simulink subsystem "ES"  (R2024a)
settings: Solver=VariableStepAuto  StartTime=0.0  StopTime=100.0  RelTol=1e-3
settings Model: DefaultTestHarness=ES_Harness1  Creator=nevil  LastModifiedBy=nevil

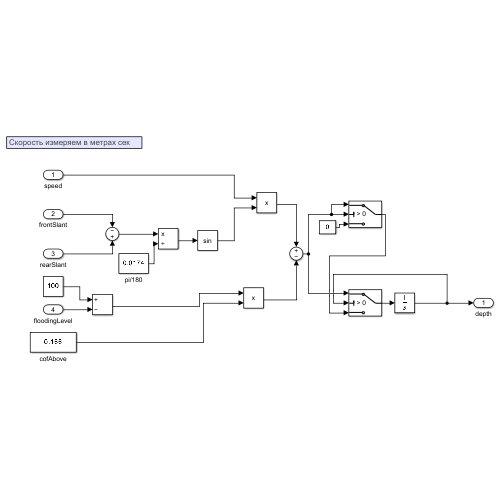
[thumbnail: Simulink's stored preview of the top-level diagram]
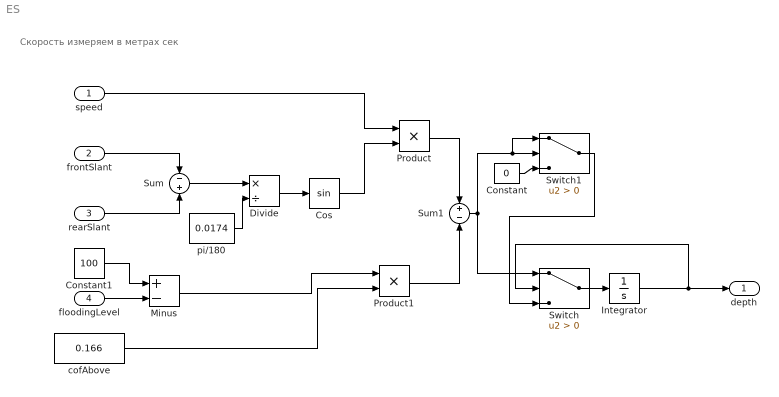
== system ES ==
  note: Скорость измеряем в метрах сек
  speed : Inport
  frontSlant : Inport  Port=2
  rearSlant : Inport  Port=3
  floodingLevel : Inport  Port=4
  Constant : Constant  Value=0
  Constant1 : Constant  Value=100
  Cos : Trigonometry
  Divide : Product  Inputs=*/
  Integrator : Integrator
  Minus : Sum  Inputs=+-
  Product : Product
  Product1 : Product
  Sum : Sum  Inputs=-|+
  Sum1 : Sum  Inputs=+|-
  Switch : Switch  Criteria=u2 > Threshold  SaturateOnIntegerOverflow=off  InputSameDT=off
  Switch1 : Switch  Criteria=u2 > Threshold  SaturateOnIntegerOverflow=off  InputSameDT=off
  cofAbove : Constant  Value=0.166
  pi/180 : Constant  Value=0.0174
  depth : Outport
  wires:
  Integrator/1 -> depth/1, Switch/2
  frontSlant/1 -> Sum/1
  rearSlant/1 -> Sum/2
  speed/1 -> Product/1
  Product/1 -> Sum1/1
  floodingLevel/1 -> Minus/2
  cofAbove/1 -> Product1/2
  Product1/1 -> Sum1/2
  Switch/1 -> Integrator/1
  Sum1/1 -> Switch1/1, Switch1/2, Switch/1
  Switch1/1 -> Switch/3
  Constant/1 -> Switch1/3
  Sum/1 -> Divide/1
  pi/180/1 -> Divide/2
  Divide/1 -> Cos/1
  Cos/1 -> Product/2
  Minus/1 -> Product1/1
  Constant1/1 -> Minus/1
